simulink model "baskModulation"  (R2021a)
settings: Solver=VariableStepAuto  StartTime=0.0  StopTime=0.5  RelTol=1e-3
undefined symbols (not defined in the file or in its folder): fdesignblkfcn, gcbh
libraries: dsparch4 x3, visionsources x1
settings Model: Creator=manami  LastModifiedBy=manami

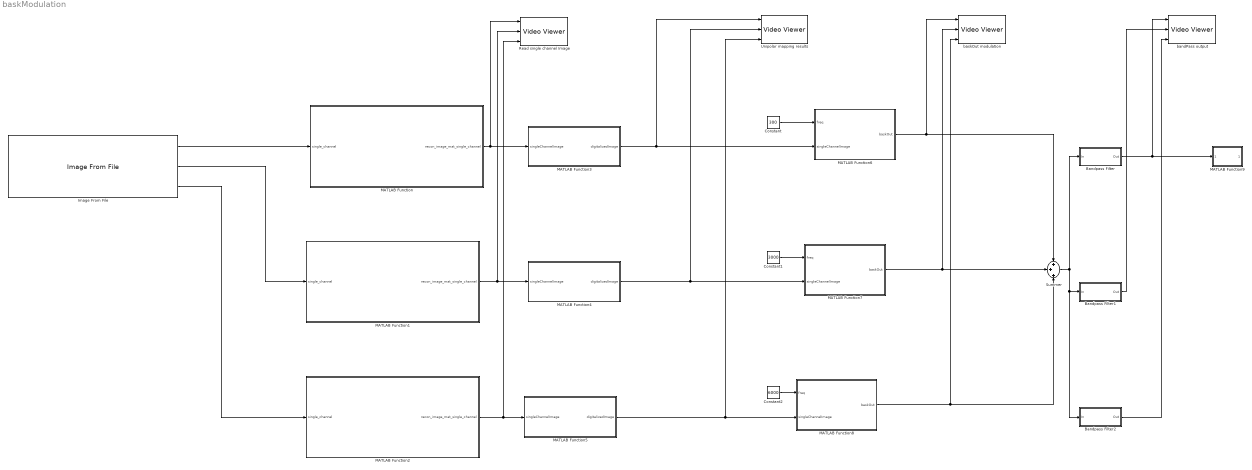
== system baskModulation ==
  Bandpass Filter : Subsystem  DialogController=fdesignblkfcn  InitFcn=fdesignblkfcn(gcbh, {'InitFcn'});  mask(Bandpass Filter){}
      mask help: Design a bandpass filter
      settings: CopyFcn=fdesignblkfcn(gcbh, {'CopyFcn'});
      mask Help: helpview(mapfilelocation('dsp'), 'dspbandpassfilter');
      mask Display: disp('Bandpass');
  Bandpass Filter1 : Subsystem  DialogController=fdesignblkfcn  InitFcn=fdesignblkfcn(gcbh, {'InitFcn'});  mask(Bandpass Filter){}
      mask help: Design a bandpass filter
      settings: CopyFcn=fdesignblkfcn(gcbh, {'CopyFcn'});
      mask Help: helpview(mapfilelocation('dsp'), 'dspbandpassfilter');
      mask Display: disp('Bandpass');
  Bandpass Filter2 : Subsystem  DialogController=fdesignblkfcn  InitFcn=fdesignblkfcn(gcbh, {'InitFcn'});  mask(Bandpass Filter){}
      mask help: Design a bandpass filter
      settings: CopyFcn=fdesignblkfcn(gcbh, {'CopyFcn'});
      mask Help: helpview(mapfilelocation('dsp'), 'dspbandpassfilter');
      mask Display: disp('Bandpass');
  Constant : Constant  Value=300
  Constant1 : Constant  Value=3000
  Constant2 : Constant  Value=6000
  Image From File : visionsources/Image From File  Tag=vipblks_nd  FileName=D:\com project\174423899_808724736692372_8447064076947490794_n.jpg  Ts=inf  imagePorts=Separate color signals  OutPortLabels=R|G|B  ImageDataType=Inherit from input image  sdImageDataType=uint(8)  Signed=on  WordLength=16  FractionLengthMode=User-defined  FractionLength=15
  MATLAB Function : MATLAB Function  TreatAsAtomicUnit=on
  MATLAB Function1 : MATLAB Function  TreatAsAtomicUnit=on
  MATLAB Function2 : MATLAB Function  TreatAsAtomicUnit=on
  MATLAB Function3 : MATLAB Function  TreatAsAtomicUnit=on
  MATLAB Function4 : MATLAB Function  TreatAsAtomicUnit=on
  MATLAB Function5 : MATLAB Function  TreatAsAtomicUnit=on
  MATLAB Function6 : MATLAB Function  TreatAsAtomicUnit=on
  MATLAB Function7 : MATLAB Function  TreatAsAtomicUnit=on
  MATLAB Function8 : MATLAB Function  TreatAsAtomicUnit=on
  MATLAB Function9 : MATLAB Function  TreatAsAtomicUnit=on
  Read single channel Image : VideoViewer  imagePorts=separate color signals  FigPos=[1 1038 1920 938]
  Summer : Sum  Inputs=+++
  Unipolar mapping results : VideoViewer  imagePorts=separate color signals  FigPos=[1 1038 1920 938]
  bandPass output : VideoViewer  imagePorts=separate color signals  FigPos=[1 1038 1920 938]
  baskOut modulation : VideoViewer  imagePorts=separate color signals  FigPos=[1 1038 1920 938]
  wires:
  Image From File/1 -> MATLAB Function/1(single_channel)
  MATLAB Function/1(recon_image_mat_single_channel) -> Read single channel Image/1, MATLAB Function3/1(singleChannelImage)
  Image From File/2 -> MATLAB Function1/1(single_channel)
  Image From File/3 -> MATLAB Function2/1(single_channel)
  MATLAB Function3/1(digitalizedImage) -> MATLAB Function6/2(singleChannelImage), Unipolar mapping results/1
  MATLAB Function4/1(digitalizedImage) -> MATLAB Function7/2(singleChannelImage), Unipolar mapping results/2
  MATLAB Function1/1(recon_image_mat_single_channel) -> Read single channel Image/2, MATLAB Function4/1(singleChannelImage)
  MATLAB Function2/1(recon_image_mat_single_channel) -> Read single channel Image/3, MATLAB Function5/1(singleChannelImage)
  MATLAB Function5/1(digitalizedImage) -> Unipolar mapping results/3, MATLAB Function8/2(singleChannelImage)
  Constant/1 -> MATLAB Function6/1(freq)
  MATLAB Function6/1(baskOut) -> Summer/1, baskOut modulation/1
  Constant1/1 -> MATLAB Function7/1(freq)
  Constant2/1 -> MATLAB Function8/1(freq)
  MATLAB Function7/1(baskOut) -> Summer/2, baskOut modulation/2
  MATLAB Function8/1(baskOut) -> Summer/3, baskOut modulation/3
  Summer/1 -> Bandpass Filter2/1(In), Bandpass Filter1/1(In), Bandpass Filter/1(In)
  Bandpass Filter/1(Out) -> MATLAB Function9/1(bandOut), bandPass output/1
  Bandpass Filter1/1(Out) -> bandPass output/2
  Bandpass Filter2/1(Out) -> bandPass output/3

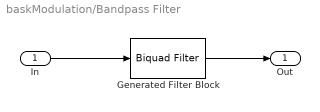
== system baskModulation/Bandpass Filter ==
  In : Inport
  Generated Filter Block : dsparch4/Biquad Filter  Tag=BlockMethodSubSystem  FilterSource=Dialog parameters  CoeffSource=Specify via dialog  FilterObject=BQF  IIRFiltStruct=Direct form II  BiQuadCoeffs=[0.0151861849028091071 0 -0.0151861849028091071 1 -1.99133602088665262 0.99265697136656994;0.00939621385102591342 0 -0.00939621385102591342 1 -1.9877444382013314 0.990133137194305069;0.00675722798635804926 0 -0.00675722798635804926 1 -1.9827668589349996 0.984699154008661925;0.00844592067035469275 0 -0.00844592067035469275 1 -1.98507595649918844 0.98733044912443757;0.00265399455961204097 0 -0.00265399455961204097 1 -1.98434855964700096 0.985971652209939653;0.0111447868027617514 0 -0.0111447868027617514 1 -1.99724083735399582 0.998489880450854184;0.0085233544999134582 0 -0.0085233544999134582 1 -1.99530240300771844 0.997845788568346825;0.00694504286439544174 0 -0.00694504286439544174 1 -1.98862750758821027 0.990023293025226292;0.0133592478822870727 0 -0.0133592478822870727 1 -1.98624373716230873 0.987740651005069803;0.00769161620716782464 0 -0.00769161620716782464 1 -1.98339842584947457 0.985496287841184704;0.003007055848346775 0 -0.003007055848346775 1 -1.98312900317526997 0.984899575957452589;0.0167442545124349973 0 -0.0167442545124349973 1 -1.99423981089542979 0.995512052389171176;2 0 -2 1 -1.99123931779938523 0.993727481915506639]  ScaleValues=[0.000265958128962854343;1;1;1;1;1;1;1;1;1;1;1;1;6.84105375107081137]  IC=0  ICnum=0  ICden=0  a0Flag=Warning  optimizeScaleValues=off  ScaleValueMode=Specify via input port (g)  InputProcessing=Columns as channels (frame based)  roundingMode=Floor  overflowMode=off  scaleValueFracLength=14  denProdOutputFracLength=30  denAccumFracLength=30  secondMemoryFracLength=15
  Out : Outport  VectorParamsAs1DForOutWhenUnconnected=off
  wires:
  In/1 -> Generated Filter Block/1
  Generated Filter Block/1 -> Out/1

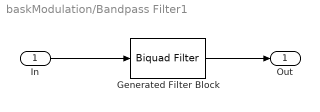
== system baskModulation/Bandpass Filter1 ==
  In : Inport
  Generated Filter Block : dsparch4/Biquad Filter  Tag=BlockMethodSubSystem  FilterSource=Dialog parameters  CoeffSource=Specify via dialog  FilterObject=BQF  IIRFiltStruct=Direct form II  BiQuadCoeffs=[0.0127638587905644918 0 -0.0127638587905644918 1 -1.81581665423310534 0.990512489891039127;0.00727410480225409994 0 -0.00727410480225409994 1 -1.80516011562094247 0.990248385680936094;0.00892100639904041225 0 -0.00892100639904041225 1 -1.80863988026950095 0.985533003680350239;0.00215213095719760713 0 -0.00215213095719760713 1 -1.80345274587490412 0.985340585386867751;0.0157885967465509133 0 -0.0157885967465509133 1 -1.82388012188242055 0.997965312187899967;0.00665989668414220231 0 -0.00665989668414220231 1 -1.81074905269629349 0.997894018640886005;0.013751788268585691 0 -0.013751788268585691 1 -1.81199133698434922 0.987613276317999667;0.00968972438386260515 0 -0.00968972438386260515 1 -1.80377057053387468 0.987349911644963218;0.00805726289477394671 0 -0.00805726289477394671 1 -1.80598589428653522 0.984415122041859991;0.00425442517540036355 0 -0.00425442517540036355 1 -1.80421325347300421 0.984344763117769972;0.0145434250343938441 0 -0.0145434250343938441 1 -1.81986654614484511 0.994039159881175749;1.21879994736572606 0 -1.21879994736572606 1 -1.80753849412703538 0.993845148244621224]  ScaleValues=[0.00388961792153109335;1;1;1;1;1;1;1;1;1;1;1;1]  IC=0  ICnum=0  ICden=0  a0Flag=Warning  optimizeScaleValues=off  ScaleValueMode=Specify via input port (g)  InputProcessing=Columns as channels (frame based)  roundingMode=Floor  overflowMode=off  scaleValueFracLength=14  denProdOutputFracLength=30  denAccumFracLength=30  secondMemoryFracLength=15
  Out : Outport  VectorParamsAs1DForOutWhenUnconnected=off
  wires:
  In/1 -> Generated Filter Block/1
  Generated Filter Block/1 -> Out/1

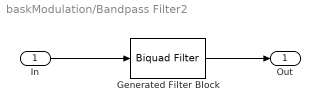
== system baskModulation/Bandpass Filter2 ==
  In : Inport
  Generated Filter Block : dsparch4/Biquad Filter  Tag=BlockMethodSubSystem  FilterSource=Dialog parameters  CoeffSource=Specify via dialog  FilterObject=BQF  IIRFiltStruct=Direct form II  BiQuadCoeffs=[0.0127129509684592787 0 -0.0127129509684592787 1 -1.31293420185322907 0.990367677319217599;0.00734466179809157172 0 -0.00734466179809157172 1 -1.29378580494437267 0.990261740578597616;0.00890518662392261046 0 -0.00890518662392261046 1 -1.30475605778007786 0.985376121752175704;0.00220758376442995157 0 -0.00220758376442995157 1 -1.29552525722728573 0.985298951502276199;0.0157846522881819815 0 -0.0157846522881819815 1 -1.3202836869756962 0.99792976740778172;0.00674222816428230072 0 -0.00674222816428230072 1 -1.29633160125723812 0.99790116630476855;0.0137422391453692096 0 -0.0137422391453692096 1 -1.30881416747602031 0.987448998243142806;0.00970163417338144873 0 -0.00970163417338144873 1 -1.29412636914199641 0.987343367152617502;0.0080801997244370205 0 -0.0080801997244370205 1 -1.30102856755786656 0.984287648878337973;0.0043656413351494212 0 -0.0043656413351494212 1 -1.29788052427160405 0.984259432231402664;0.0144781777770884301 0 -0.0144781777770884301 1 -1.31684388478308589 0.993939602985425497;0.664800736901837941 0 -0.664800736901837941 1 -1.29453521410102246 0.993861775273674919]  ScaleValues=[0.00724341532381073561;1;1;1;1;1;1;1;1;1;1;1;1]  IC=0  ICnum=0  ICden=0  a0Flag=Warning  optimizeScaleValues=off  ScaleValueMode=Specify via input port (g)  InputProcessing=Columns as channels (frame based)  roundingMode=Floor  overflowMode=off  scaleValueFracLength=14  denProdOutputFracLength=30  denAccumFracLength=30  secondMemoryFracLength=15
  Out : Outport  VectorParamsAs1DForOutWhenUnconnected=off
  wires:
  In/1 -> Generated Filter Block/1
  Generated Filter Block/1 -> Out/1

== matlab function baskModulation/MATLAB Function ==
  data: single_channel input; recon_image_mat_single_channel output
function recon_image_mat_single_channel = single_channel_image_read(single_channel)
%#codegen
row = length(single_channel(:,1));
col = length(single_channel);
bin = zeros(1,row*col);;
k=1;
for i=1:row
    bin(1,k:k+col-1) = single_channel(i,:);
    k = k+col;
end
binla = dec2bin(bin);
bintemp = binla;
bintemp(:,7:8) = '0';
new = bin2dec(bintemp)';
recon = zeros(row,col);
for i = 1:row
    recon(i,1:col) = new(1,col*(i-1)+1:col*i);
end 
newimage = recon;
recon_image_mat_single_channel = cast(newimage,'uint8');

== matlab function baskModulation/MATLAB Function2 ==
  data: single_channel input; recon_image_mat_single_channel output
function recon_image_mat_single_channel = single_channel_image_read(single_channel)
%#codegen
row = length(single_channel(:,1));
col = length(single_channel);
bin = zeros(1,row*col);;
k=1;
for i=1:row
    bin(1,k:k+col-1) = single_channel(i,:);
    k = k+col;
end
binla = dec2bin(bin);
bintemp = binla;
bintemp(:,7:8) = '0';
new = bin2dec(bintemp)';
recon = zeros(row,col);
for i = 1:row
    recon(i,1:col) = new(1,col*(i-1)+1:col*i);
end 
newimage = recon;
recon_image_mat_single_channel = cast(newimage,'uint8');

== matlab function baskModulation/MATLAB Function3 ==
  data: singleChannelImage input; digitalizedImage output
function digitalizedImage = unipolar_mapping(singleChannelImage)
imageShape = size(singleChannelImage);
threshold = mean(singleChannelImage, 'all');
N = imageShape(2) % N = input size
% n = image row

% Unipolar mapping
for indImg = 1:imageShape(1)
    for i = 1:N
        if singleChannelImage(indImg, i)<=threshold
            singleChannelImage(indImg, i) = 0;
        else
            singleChannelImage(indImg, i) = 255;
        end          
    end
end
digitalizedImage = singleChannelImage;

%NOTE: we have used the mean pixel as threshold for unipolar mapping
%NOTE: I do not need the continuous assigning variable thing for now, if I
%this, the quality will be better, we will keep this for later
%NOTE: Single Channel Image Dim 1932*2576

== matlab function baskModulation/MATLAB Function4 ==
  data: singleChannelImage input; digitalizedImage output
function digitalizedImage = unipolar_mapping(singleChannelImage)
imageShape = size(singleChannelImage);
threshold = mean(singleChannelImage, 'all');
N = imageShape(2) % N = input size
% n = image row

% Unipolar mapping
for indImg = 1:imageShape(1)
    for i = 1:N
        if singleChannelImage(indImg, i)<=threshold
            singleChannelImage(indImg, i) = 0;
        else
            singleChannelImage(indImg, i) = 255;
        end          
    end
end
digitalizedImage = singleChannelImage;

== matlab function baskModulation/MATLAB Function5 ==
  data: singleChannelImage input; digitalizedImage output
function digitalizedImage = unipolar_mapping(singleChannelImage)
imageShape = size(singleChannelImage);
threshold = mean(singleChannelImage, 'all');
N = imageShape(2) % N = input size
% n = image row

% Unipolar mapping
for indImg = 1:imageShape(1)
    for i = 1:N
        if singleChannelImage(indImg, i)<=threshold
            singleChannelImage(indImg, i) = 0;
        else
            singleChannelImage(indImg, i) = 255;
        end          
    end
end
digitalizedImage = singleChannelImage;

== matlab function baskModulation/MATLAB Function6 ==
  data: freq input; baskOut output; singleChannelImage input
function baskOut = bask_signal(freq, singleChannelImage)
sizeIm = size(singleChannelImage)
baskOut = zeros(sizeIm)
carrier = cos(2*pi*freq*sizeIm(2))
% for i = 1: sizeIm(1)
%     baskOut(i, :) = singleChannelImage(i, :).*carrier
% end
baskOut(:, :) = singleChannelImage.*carrier
baskOut = baskOut;

== matlab function baskModulation/MATLAB Function7 ==
  data: freq input; baskOut output; singleChannelImage input
function baskOut = bask_signal(freq, singleChannelImage)
sizeIm = size(singleChannelImage)
baskOut = zeros(sizeIm)
carrier = cos(2*pi*freq*sizeIm(2))
% for i = 1: sizeIm(1)
%     baskOut(i, :) = singleChannelImage(i, :).*carrier
% end
baskOut(:, :) = singleChannelImage.*carrier
baskOut = baskOut;

== matlab function baskModulation/MATLAB Function8 ==
  data: freq input; baskOut output; singleChannelImage input
function baskOut = bask_signal(freq, singleChannelImage)
sizeIm = size(singleChannelImage)
baskOut = zeros(sizeIm)
carrier = cos(2*pi*freq*sizeIm(2))
% for i = 1: sizeIm(1)
%     baskOut(i, :) = singleChannelImage(i, :).*carrier
% end
baskOut(:, :) = singleChannelImage.*carrier
baskOut = baskOut;

== matlab function baskModulation/MATLAB Function9 ==
  data: bandOut input; deModulated output
function deModulated = productModulation(bandOut)


deModulated = bandOut

== matlab function baskModulation/MATLAB Function1 ==
  data: single_channel input; recon_image_mat_single_channel output
function recon_image_mat_single_channel = single_channel_image_read(single_channel)
%#codegen
row = length(single_channel(:,1));
col = length(single_channel);
bin = zeros(1,row*col);;
k=1;
for i=1:row
    bin(1,k:k+col-1) = single_channel(i,:);
    k = k+col;
end
binla = dec2bin(bin);
bintemp = binla;
bintemp(:,7:8) = '0';
new = bin2dec(bintemp)';
recon = zeros(row,col);
for i = 1:row
    recon(i,1:col) = new(1,col*(i-1)+1:col*i);
end 
newimage = recon;
recon_image_mat_single_channel = cast(newimage,'uint8');
